simulink model "ParallelForce"  (R2022b)
settings: Solver=VariableStepAuto  StartTime=0.0  StopTime=5  RelTol=1e-3
values from neighbouring files (symbols this model uses):
  fd = [0,0,3,0,0,0]    [parameters.m]
  Kd = diag([25,25,25,1,1,1])    [parameters.m]
  Kf = diag([55,55,55,1,1,1])    [parameters.m]
  Ki = diag([50,50,50,1,1,1])    [parameters.m]
  Kp = diag([40,40,40,1,1,1])    [parameters.m]
  Md = diag([0.12,0.12,0.12,0,0,0])    [parameters.m]
  xd = [H(1:3,4); eulers']    [parameters.m]
undefined symbols (not defined in the file or in its folder): parms
settings Model: Creator=uzair  LastModifiedBy=uzair

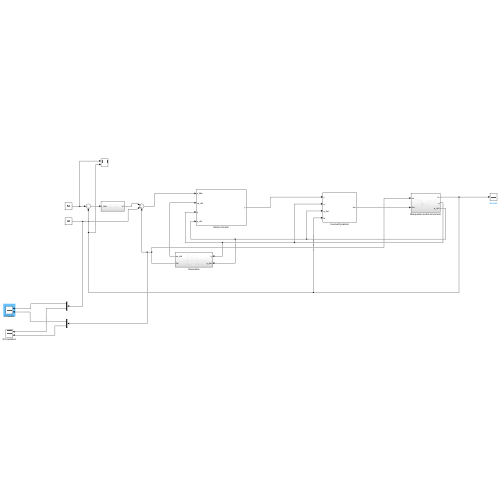
[thumbnail: Simulink's stored preview of the top-level diagram]
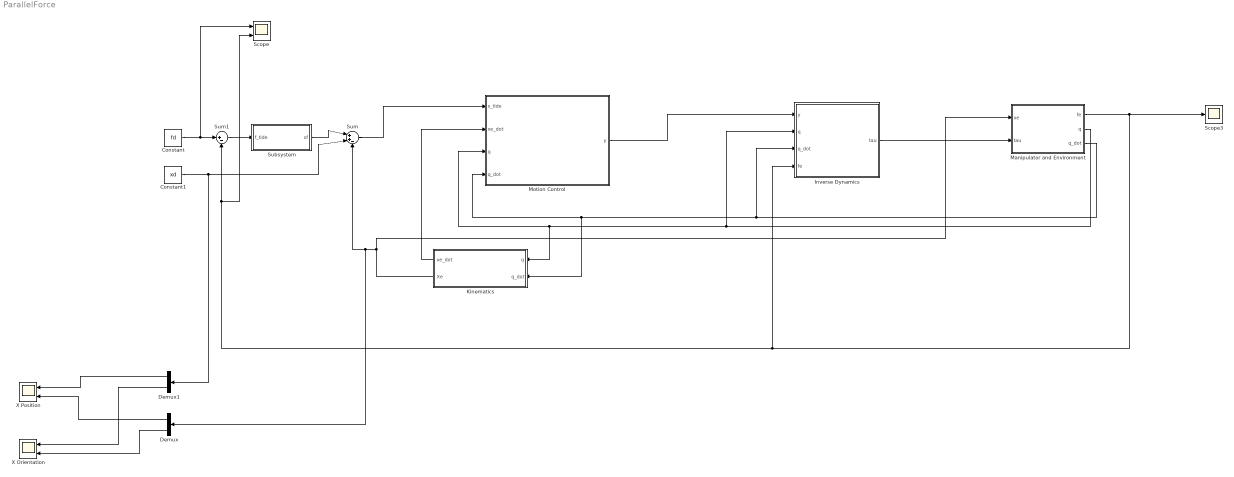
== system ParallelForce ==
  Constant : Constant  Value=fd
  Constant1 : Constant  Value=xd
  Demux : Demux  Outputs=2
  Demux1 : Demux  Outputs=2
  Inverse Dynamics : Subsystem
  Kinematics : Subsystem
  Manipulator and Environment : Subsystem
  Motion Control : Subsystem
  Scope : Scope  NumInputPorts=2
  Scope3 : Scope
  Subsystem : Subsystem
  Sum : Sum  Inputs=|++-
  Sum1 : Sum  Inputs=|+-
  X Orientation : Scope  NumInputPorts=2
  X Position : Scope  NumInputPorts=2
  wires:
  Motion Control/1(y) -> Inverse Dynamics/1(y)
  Kinematics/2(Xe) -> Demux/1, Sum/3, Manipulator and Environment/1(xe)
  Kinematics/1(xe_dot) -> Motion Control/2(xe_dot)
  Manipulator and Environment/2(q) -> Inverse Dynamics/2(q), Kinematics/1(q), Motion Control/3(q)
  Manipulator and Environment/3(q_dot) -> Inverse Dynamics/3(q_dot), Kinematics/2(q_dot), Motion Control/4(q_dot)
  Manipulator and Environment/1(fe) -> Scope3/1, Sum1/2, Scope/2, Inverse Dynamics/4(fe)
  Inverse Dynamics/1(tau) -> Manipulator and Environment/2(tau)
  Sum/1 -> Motion Control/1(x_tide)
  Subsystem/1(xf) -> Sum/1
  Constant/1 -> Scope/1, Sum1/1
  Sum1/1 -> Subsystem/1(f_tide)
  Constant1/1 -> Demux1/1, Sum/2
  Demux/2 -> X Orientation/2
  Demux/1 -> X Position/2
  Demux1/2 -> X Orientation/1
  Demux1/1 -> X Position/1

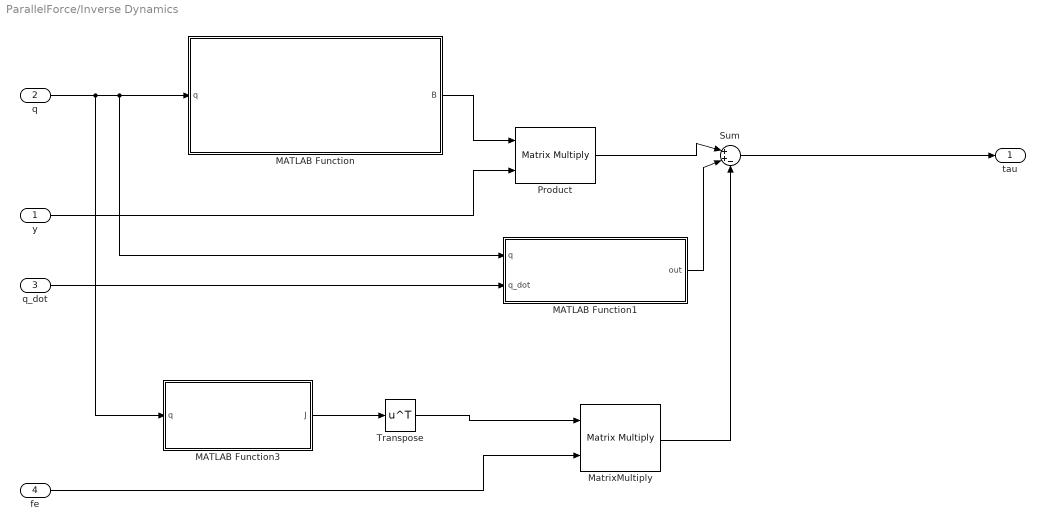
== system ParallelForce/Inverse Dynamics ==
  y : Inport
  q : Inport  Port=2
  q_dot : Inport  Port=3
  fe : Inport  Port=4
  MATLAB Function : MATLAB Function  TreatAsAtomicUnit=on
  MATLAB Function1 : MATLAB Function  TreatAsAtomicUnit=on
  MATLAB Function3 : MATLAB Function  TreatAsAtomicUnit=on
  MatrixMultiply : Product  Multiplication=Matrix(*)
  Product : Product  Multiplication=Matrix(*)
  Sum : Sum  Inputs=|++-
  Transpose : Math  Operator=transpose  OutputSignalType=real
  tau : Outport
  wires:
  q/1 -> MATLAB Function3/1(q), MATLAB Function1/1(q), MATLAB Function/1(q)
  MATLAB Function/1(B) -> Product/1
  y/1 -> Product/2
  q_dot/1 -> MATLAB Function1/2(q_dot)
  MATLAB Function1/1(out) -> Sum/2
  Sum/1 -> tau/1
  MATLAB Function3/1(J) -> Transpose/1
  fe/1 -> MatrixMultiply/2
  Transpose/1 -> MatrixMultiply/1
  MatrixMultiply/1 -> Sum/3
  Product/1 -> Sum/1

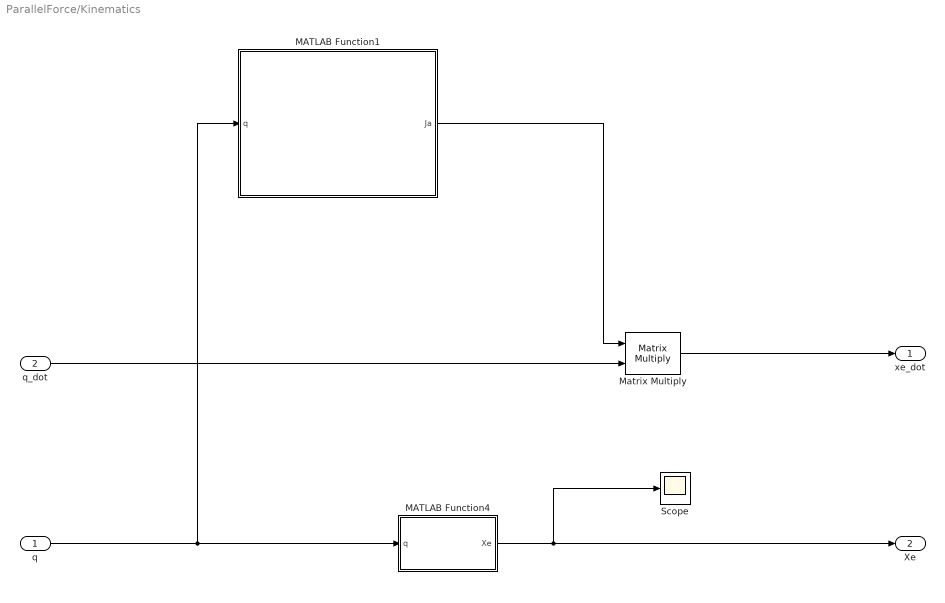
== system ParallelForce/Kinematics ==
  q : Inport
  q_dot : Inport  Port=2
  MATLAB Function1 : MATLAB Function  TreatAsAtomicUnit=on
  MATLAB Function4 : MATLAB Function  TreatAsAtomicUnit=on
  Matrix Multiply : Product  Multiplication=Matrix(*)
  Scope : Scope
  xe_dot : Outport
  Xe : Outport  Port=2
  wires:
  MATLAB Function1/1(Ja) -> Matrix Multiply/1
  q/1 -> MATLAB Function1/1(q), MATLAB Function4/1(q)
  MATLAB Function4/1(Xe) -> Scope/1, Xe/1
  Matrix Multiply/1 -> xe_dot/1
  q_dot/1 -> Matrix Multiply/2

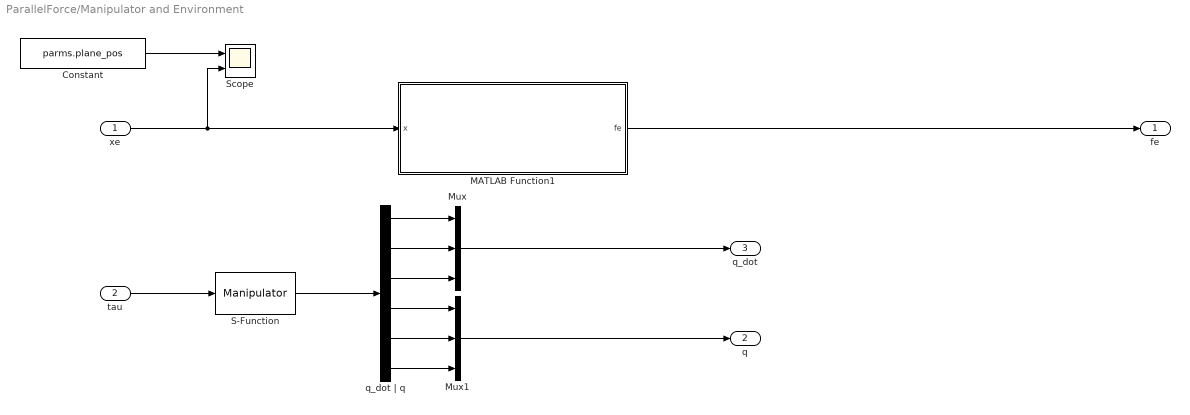
== system ParallelForce/Manipulator and Environment ==
  xe : Inport
  tau : Inport  Port=2
  Constant : Constant  Value=parms.plane_pos
  MATLAB Function1 : MATLAB Function  TreatAsAtomicUnit=on
  Mux : Mux  Inputs=3
  Mux1 : Mux  Inputs=3
  S-Function : S-Function  FunctionName=Manipulator  Parameters=params  SFunctionDeploymentMode=off  EnableBusSupport=off
  Scope : Scope  NumInputPorts=2
  q_dot | q : Demux  Outputs=6
  fe : Outport
  q : Outport  Port=2
  q_dot : Outport  Port=3
  wires:
  MATLAB Function1/1(fe) -> fe/1
  S-Function/1 -> q_dot | q/1
  q_dot | q/4 -> Mux1/1
  q_dot | q/1 -> Mux/1
  q_dot | q/6 -> Mux1/3
  q_dot | q/2 -> Mux/2
  q_dot | q/5 -> Mux1/2
  q_dot | q/3 -> Mux/3
  Mux/1 -> q_dot/1
  Mux1/1 -> q/1
  tau/1 -> S-Function/1
  Constant/1 -> Scope/1
  xe/1 -> Scope/2, MATLAB Function1/1(x)

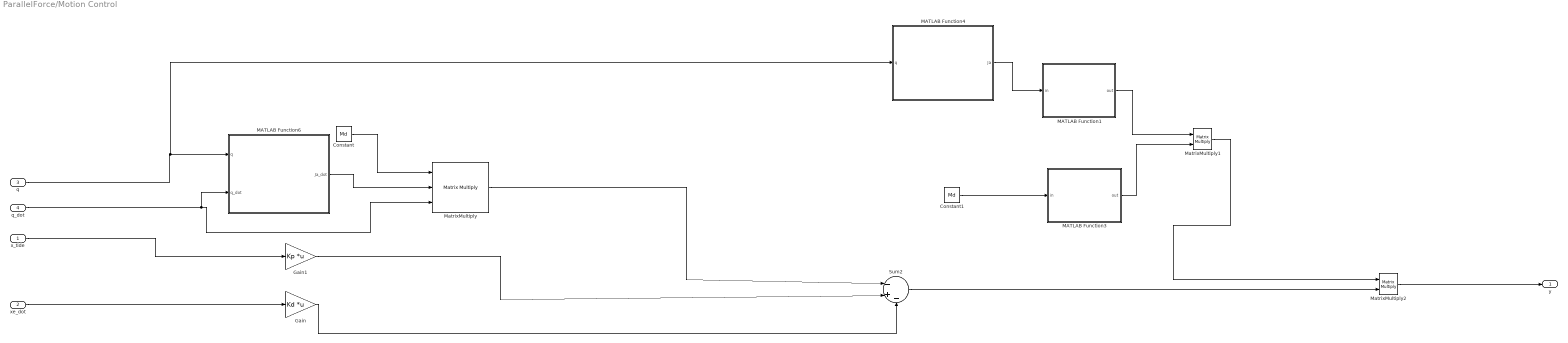
== system ParallelForce/Motion Control ==
  x_tide : Inport
  xe_dot : Inport  Port=2
  q : Inport  Port=3
  q_dot : Inport  Port=4
  Constant : Constant  Value=Md  VectorParams1D=off
  Constant1 : Constant  Value=Md  VectorParams1D=off
  Gain : Gain  Gain=Kd  Multiplication=Matrix(K*u)
  Gain1 : Gain  Gain=Kp  Multiplication=Matrix(K*u)
  MATLAB Function1 : MATLAB Function  TreatAsAtomicUnit=on
  MATLAB Function3 : MATLAB Function  TreatAsAtomicUnit=on
  MATLAB Function4 : MATLAB Function  TreatAsAtomicUnit=on
  MATLAB Function6 : MATLAB Function  TreatAsAtomicUnit=on
  MatrixMultiply : Product  Inputs=3  Multiplication=Matrix(*)
  MatrixMultiply1 : Product  Multiplication=Matrix(*)
  MatrixMultiply2 : Product  Multiplication=Matrix(*)
  Sum2 : Sum  Inputs=|-+-
  y : Outport
  wires:
  q/1 -> MATLAB Function4/1(q), MATLAB Function6/1(q)
  q_dot/1 -> MATLAB Function6/2(q_dot), MatrixMultiply/3
  Constant/1 -> MatrixMultiply/1
  MATLAB Function6/1(Ja_dot) -> MatrixMultiply/2
  MATLAB Function1/1(out) -> MatrixMultiply1/1
  MATLAB Function3/1(out) -> MatrixMultiply1/2
  MATLAB Function4/1(Ja) -> MATLAB Function1/1(in)
  Constant1/1 -> MATLAB Function3/1(in)
  Sum2/1 -> MatrixMultiply2/2
  MatrixMultiply1/1 -> MatrixMultiply2/1
  MatrixMultiply2/1 -> y/1
  xe_dot/1 -> Gain/1
  x_tide/1 -> Gain1/1
  MatrixMultiply/1 -> Sum2/1
  Gain/1 -> Sum2/3
  Gain1/1 -> Sum2/2

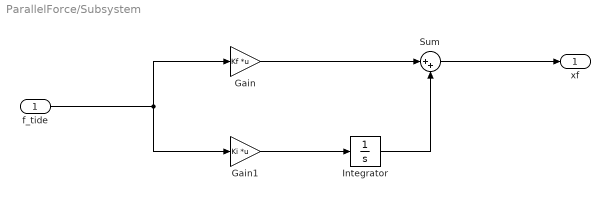
== system ParallelForce/Subsystem ==
  f_tide : Inport
  Gain : Gain  Gain=Kf  Multiplication=Matrix(K*u)
  Gain1 : Gain  Gain=Ki  Multiplication=Matrix(K*u)
  Integrator : Integrator
  Sum : Sum  Inputs=|++
  xf : Outport
  wires:
  f_tide/1 -> Gain1/1, Gain/1
  Gain1/1 -> Integrator/1
  Integrator/1 -> Sum/2
  Gain/1 -> Sum/1
  Sum/1 -> xf/1

== matlab function ParallelForce/Inverse Dynamics/MATLAB Function1 ==
  data: q input; out output; q_dot input; params parameter
function out = n(q, q_dot, params)
    
    m1 = params.m(1);
    m2 = params.m(2);
    m3 = params.m(3);

    q1 = q(1);
    q2 = q(2);
    q3 = q(3);

    q1_dot = q_dot(1);
    q2_dot = q_dot(2);
    q3_dot = q_dot(3);

    g = params.g;

    Fv = params.Fv;
 

    C = [[q2_dot*((3*m2)/20 + (3*m3)/10 + m2*q2 + m3*q2) - q3_dot*((4*m3*sin(2*q3))/625 + (4*m3*sin(q3))/125), q1_dot*((3*m2)/20 + (3*m3)/10 + m2*q2 + m3*q2), (2*m3*q3_dot*cos(q3)*(q2 + 3/10))/25 - q1_dot*((4*m3*sin(q3))/125 + (8*m3*cos(q3)*sin(q3))/625)]
        [                        -q1_dot*((3*m2)/20 + (3*m3)/10 + m2*q2 + m3*q2) - (2*m3*q3_dot*sin(q3))/25,                                              0,                                                                       -(2*m3*q1_dot*sin(q3))/25]
        [                      q1_dot*((4*m3*sin(2*q3))/625 + (4*m3*sin(q3))/125) + (2*m3*q2_dot*sin(q3))/25,                       (2*m3*q1_dot*sin(q3))/25,                                                                                               0]];

    G = [(g*m1*cos(q1))/5 - g*m2*((3*sin(q1))/20 - (2*cos(q1))/5 + q2*sin(q1)) + g*m3*((2*cos(q1))/5 + (2*cos(q1)*cos(q3))/25 - sin(q1)*(q2 + 3/10));
                                                                                                                        g*cos(q1)*(m2 + m3);
                                                                                                               -(2*g*m3*sin(q1)*sin(q3))/25];

    out = C*q_dot + diag(Fv)*q_dot + G;
end

== matlab function ParallelForce/Inverse Dynamics/MATLAB Function ==
  data: q input; B output; params parameter
function B = inertiaMatrix(q, params)
    q1 = q(1); % not used in this matrix
    q2 = q(2);
    q3 = q(3);

    m1 = params.m(1);
    m2 = params.m(2);
    m3 = params.m(3);

    B = [[(195791581307*m1)/1220703125000 + (8503*m2)/40000 + (321279862557*m3)/1220703125000 + (8*m3*cos(q3)^2)/625 + (3*m2*q2)/10 + (3*m3*q2)/5 + m2*q2^2 + m3*q2^2 + (8*m3*cos(q3))/125, (2*m2)/5 + (2*m3)/5 + (2*m3*cos(q3))/25, (2*m3*sin(q3)*(q2 + 3/10))/25]
        [                                                                                                                                         (2*m2)/5 + (2*m3)/5 + (2*m3*cos(q3))/25,                                 m2 + m3,                             0]
        [                                                                                                                                                   (2*m3*sin(q3)*(q2 + 3/10))/25,                                       0,            (32637*m3)/1562500]];
end

== matlab function ParallelForce/Kinematics/MATLAB Function4 ==
  data: q input; Xe output
function Xe = Kinematics(q)
    q1 = q(1);
    q2 = q(2);
    q3 = q(3);
    
    H = [[       0,         -cos(q3),        -sin(q3),                                                     -(4*sin(q3))/25]
         [ sin(q1), -cos(q1)*sin(q3), cos(q1)*cos(q3),        (2*cos(q1))/5 + (4*cos(q1)*cos(q3))/25 - sin(q1)*(q2 + 3/10)]
         [-cos(q1), -sin(q1)*sin(q3), cos(q3)*sin(q1), (2*sin(q1))/5 + cos(q1)*(q2 + 3/10) + (4*cos(q3)*sin(q1))/25 + 3/20]
         [       0,                0,               0,                                                                   1]];


    eulers = rotm2eul(H(1:3,1:3), "ZYZ");

    Xe = [H(1:3,4); eulers'];
end

== matlab function ParallelForce/Motion Control/MATLAB Function1 ==
  data: in input; out output
function out = inv(in)
    out = pinv(in);
end

== matlab function ParallelForce/Kinematics/MATLAB Function1 ==
  data: q input; Ja output
function Ja = AnalyticalJacobian(q)
    q1 = q(1);
    q2 = q(2);
    q3 = q(3);

    H = [[       0,         -cos(q3),        -sin(q3),                                                     -(4*sin(q3))/25]
[ sin(q1), -cos(q1)*sin(q3), cos(q1)*cos(q3),        (2*cos(q1))/5 + (4*cos(q1)*cos(q3))/25 - sin(q1)*(q2 + 3/10)]
[-cos(q1), -sin(q1)*sin(q3), cos(q3)*sin(q1), (2*sin(q1))/5 + cos(q1)*(q2 + 3/10) + (4*cos(q3)*sin(q1))/25 + 3/20]
[       0,                0,               0,                                                                   1]];


eulers = rotm2eul(H(1:3,1:3), "ZYZ");


    phi1 = eulers(1);
    phi2 = eulers(2);
    phi3 = eulers(3); %not used

Ja_m = [
[                                                             0,        0,                                             -(4*cos(q3))/25]
[- (2*sin(q1))/5 - cos(q1)*(q2 + 3/10) - (4*cos(q3)*sin(q1))/25, -sin(q1),                                     -(4*cos(q1)*sin(q3))/25]
[  (2*cos(q1))/5 + (4*cos(q1)*cos(q3))/25 - sin(q1)*(q2 + 3/10),  cos(q1),                                     -(4*sin(q1)*sin(q3))/25]
[                              -(cos(phi1)*cos(phi2))/sin(phi2),        0, (cos(q1)*sin(phi2) + cos(phi2)*sin(phi1)*sin(q1))/sin(phi2)]
[                                                    -sin(phi1),        0,                                          -cos(phi1)*sin(q1)]
[                                           cos(phi1)/sin(phi2),        0,                              -(sin(phi1)*sin(q1))/sin(phi2)]
];


    Ja = Ja_m;
end

== matlab function ParallelForce/Manipulator and Environment/MATLAB Function1 ==
  data: x input; fe output; parms parameter
function fe = Environment(x, parms)
    if(x(parms.plane_axis) >= parms.plane_pos(parms.plane_axis))
        xr = parms.plane_pos;

        xe = zeros(6,1);
        xe(parms.plane_axis) = x(parms.plane_axis);

        fe = parms.Ke * (xe - xr);

    else
        fe = zeros(6,1);
    end
end

== matlab function ParallelForce/Motion Control/MATLAB Function3 ==
  data: in input; out output
function out = inv(in)
    out = pinv(in);
end

== matlab function ParallelForce/Motion Control/MATLAB Function4 ==
  data: q input; Ja output
function Ja = AnalyticalJacobian(q)
    
    q1 = q(1);
    q2 = q(2);
    q3 = q(3);

       H = [[       0,         -cos(q3),        -sin(q3),                                                     -(4*sin(q3))/25]
         [ sin(q1), -cos(q1)*sin(q3), cos(q1)*cos(q3),        (2*cos(q1))/5 + (4*cos(q1)*cos(q3))/25 - sin(q1)*(q2 + 3/10)]
         [-cos(q1), -sin(q1)*sin(q3), cos(q3)*sin(q1), (2*sin(q1))/5 + cos(q1)*(q2 + 3/10) + (4*cos(q3)*sin(q1))/25 + 3/20]
         [       0,                0,               0,                                                                   1]];


        eulers = rotm2eul(H(1:3,1:3), "ZYZ");


        phi1 = eulers(1);
        phi2 = eulers(2);
        phi3 = eulers(3); %not used

        Ja = [
               [                                                                     0,        0,                                             -(4*cos(q3))/25]
               [- (3*cos(q1))/10 - (2*sin(q1))/5 - (4*cos(q3)*sin(q1))/25 - q2*cos(q1), -sin(q1),                                     -(4*cos(q1)*sin(q3))/25]
               [  (2*cos(q1))/5 - (3*sin(q1))/10 + (4*cos(q1)*cos(q3))/25 - q2*sin(q1),  cos(q1),                                     -(4*sin(q1)*sin(q3))/25]
               [                                      -(cos(phi1)*cos(phi2))/sin(phi2),        0, (cos(q1)*sin(phi2) + cos(phi2)*sin(phi1)*sin(q1))/sin(phi2)]
               [                                                            -sin(phi1),        0,                                          -cos(phi1)*sin(q1)]
               [                                                   cos(phi1)/sin(phi2),        0,                              -(sin(phi1)*sin(q1))/sin(phi2)]];

end

== matlab function ParallelForce/Inverse Dynamics/MATLAB Function3 ==
  data: q input; J output
function J = GeomatricalJacobian(q)
q1 = q(1);
q2 = q(2);
q3 = q(3);

    J = [
[                                                             0,        0,         -(4*cos(q3))/25]
[- (2*sin(q1))/5 - cos(q1)*(q2 + 3/10) - (4*cos(q3)*sin(q1))/25, -sin(q1), -(4*cos(q1)*sin(q3))/25]
[  (2*cos(q1))/5 + (4*cos(q1)*cos(q3))/25 - sin(q1)*(q2 + 3/10),  cos(q1), -(4*sin(q1)*sin(q3))/25]
[                                                             1,        0,                       0]
[                                                            0,        0,                -sin(q1)]
[                                                             0,        0,                 cos(q1)]];

end

== matlab function ParallelForce/Motion Control/MATLAB Function6 ==
  data: q input; Ja_dot output; q_dot input
function Ja_dot = AnalyticalJacobian_Dot(q, q_dot)
q1 = q(1);
q2 = q(2);
q3 = q(3);

q1_dot = q_dot(1);
q2_dot = q_dot(2);
q3_dot = q_dot(3);

H = [[       0,         -cos(q3),        -sin(q3),                                                     -(4*sin(q3))/25]
[ sin(q1), -cos(q1)*sin(q3), cos(q1)*cos(q3),        (2*cos(q1))/5 + (4*cos(q1)*cos(q3))/25 - sin(q1)*(q2 + 3/10)]
[-cos(q1), -sin(q1)*sin(q3), cos(q3)*sin(q1), (2*sin(q1))/5 + cos(q1)*(q2 + 3/10) + (4*cos(q3)*sin(q1))/25 + 3/20]
[       0,                0,               0,                                                                   1]];



eulers = rotm2eul(H(1:3,1:3), "ZYZ");


phi1 = eulers(1);
phi2 = eulers(2);
phi3 = eulers(3); %not used

Ja_dot_m = [
[                                                                                                                                   0,               0,                                                 (4*q3_dot*sin(q3))/25]
[  q1_dot*sin(q1)*(q2 + 3/10) - q2_dot*cos(q1) - (4*q1_dot*cos(q1)*cos(q3))/25 - (2*q1_dot*cos(q1))/5 + (4*q3_dot*sin(q1)*sin(q3))/25, -q1_dot*cos(q1),         (4*q1_dot*sin(q1)*sin(q3))/25 - (4*q3_dot*cos(q1)*cos(q3))/25]
[- (2*q1_dot*sin(q1))/5 - q2_dot*sin(q1) - q1_dot*cos(q1)*(q2 + 3/10) - (4*q1_dot*cos(q3)*sin(q1))/25 - (4*q3_dot*cos(q1)*sin(q3))/25, -q1_dot*sin(q1),       - (4*q1_dot*cos(q1)*sin(q3))/25 - (4*q3_dot*cos(q3)*sin(q1))/25]
[                                                                                                                                   0,               0, -(q1_dot*(sin(phi2)*sin(q1) - cos(phi2)*cos(q1)*sin(phi1)))/sin(phi2)]
[                                                                                                                                   0,               0,                                             -q1_dot*cos(phi1)*cos(q1)]
[                                                                                                                                   0,               0,                                 -(q1_dot*cos(q1)*sin(phi1))/sin(phi2)]
];

Ja_dot = Ja_dot_m;
end
